simulink model "dq0_fun"  (R2020b)
settings: Solver=FixedStepAuto  StartTime=0.0  StopTime=0.25  FixedStep=1e-3  RelTol=1e-3
libraries: powerlib x13, powerlib_meascontrol x2
settings Model: Creator=kacper  LastModifiedBy=kacper

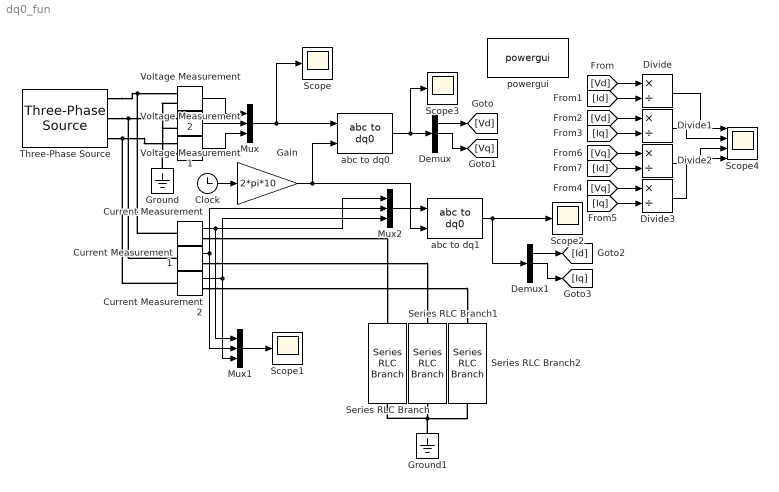
== system dq0_fun ==
  Clock : Clock
  Current Measurement : powerlib/Measurements/Current Measurement  PhasorSimulation=off  OutputType=Complex  PSBequivalent=0
  Current Measurement1 : powerlib/Measurements/Current Measurement  PhasorSimulation=off  OutputType=Complex  PSBequivalent=0
  Current Measurement2 : powerlib/Measurements/Current Measurement  PhasorSimulation=off  OutputType=Complex  PSBequivalent=0
  Demux : Demux  Outputs=3
  Demux1 : Demux  Outputs=3
  Divide{,1..3} (4 alike) : Product  Inputs=*/
  Gain : Gain  Gain=2*pi*10
  Ground : powerlib/Elements/Ground  LConnTagsString=a
  Ground1 : powerlib/Elements/Ground  LConnTagsString=a
  Mux : Mux  Inputs=3
  Mux1 : Mux  Inputs=3
  Mux2 : Mux  Inputs=3
  Scope{,1..3} (4 alike) : Scope
  Scope4 : Scope  NumInputPorts=4
  Series RLC Branch : powerlib/Elements/Series RLC Branch  LConnTagsString=__new0  RConnTagsString=__new0  BranchType=R  Resistance=1  Inductance=1e-3  SetiL0=off  InitialCurrent=0  Capacitance=1e-6  Setx0=off  InitialVoltage=0  Measurements=None
  Series RLC Branch1 : powerlib/Elements/Series RLC Branch  LConnTagsString=__new0  RConnTagsString=__new0  BranchType=L  Resistance=1  Inductance=1  SetiL0=off  InitialCurrent=0  Capacitance=1e-6  Setx0=off  InitialVoltage=0  Measurements=None
  Series RLC Branch2 : powerlib/Elements/Series RLC Branch  LConnTagsString=__new0  RConnTagsString=__new0  BranchType=R  Resistance=1  Inductance=1  SetiL0=off  InitialCurrent=0  Capacitance=1e-6  Setx0=off  InitialVoltage=0  Measurements=None
  Three-Phase Source : powerlib/Electrical Sources/Three-Phase Source  InternalConnection=Yg  VoltagePhases=on  Voltage=1/sqrt(2)  PhaseAngle=0  Voltage_phases=[1/sqrt(2) 1/sqrt(2) 1/sqrt(2)]  PhaseAngles_phases=[0 -120 +120]  Frequency=50  NonIdealSource=off  SpecifyImpedance=off  Resistance=0.8929  Inductance=16.58e-3  ShortCircuitLevel=100e6  BaseVoltage=25e3  XRratio=7  BusType=swing  Pref=10e3  Qref=0  Prefabc=[10e3, 10e3, 10e3]  Qrefabc=[0, 0, 0]  Qmin=-inf  Qmax=inf
  Voltage Measurement : powerlib/Measurements/Voltage Measurement  PhasorSimulation=off  OutputType=Complex  PSBequivalent=0
  Voltage Measurement1 : powerlib/Measurements/Voltage Measurement  PhasorSimulation=off  OutputType=Complex  PSBequivalent=0
  Voltage Measurement2 : powerlib/Measurements/Voltage Measurement  PhasorSimulation=off  OutputType=Complex  PSBequivalent=0
  abc to dq0 : powerlib_meascontrol/Transformations/abc to dq0  Alignment=90 degrees behind phase A axis
  abc to dq1 : powerlib_meascontrol/Transformations/abc to dq0  Alignment=90 degrees behind phase A axis
  powergui : powerlib/powergui  Priority=1  SimulationMode=Continuous  SampleTime=50e-6  frequency=60  Iterations=50  frequencyindice=10  Pbase=100e6  ErrMax=1e-4  UnitsV=kV  UnitsW=MW  buscounter=0  FunctionMessages=off  echomessages=off  EnableUseOfTLC=off  CurrentSourceSwitches=off  DisableSnubberDevices=off  DisableRonSwitches=off  DisableVfSwitches=off  DisplayEquations=off  AutomaticDiscreteSolvers=off  SolverType=Tustin/Backward Euler (TBE)  Interpol=off  ExternalGateDelay=off  methode=off  Ts=100  x0status=blocks  SPID=on  SwTol=0  HookPort=off  NonlinearTolerance=1e-4  nMaxIteration=100  ContinueOnMaxIteration=off  RestoreLinks=warning  ResistiveCurrentMeasurement=off  Frange=[0:2:500]  Ylog=off  Xlog=on  ShowGrid=off  save=off  variable=ZData  structure=0  ZoomFFT=off  StartTime=0.0  cycles=1  DisplayStyle=1  fundamental=60  FreqAxis=off  MaxFrequency=1000  frequencyindicesteady=1  RmsSteady=1  display=off
  wires:
  Voltage Measurement1/1 -> Mux/2
  Voltage Measurement/1 -> Mux/1
  Voltage Measurement2/1 -> Mux/3
  Mux/1 -> Scope/1, abc to dq0/1
  Clock/1 -> Gain/1
  Gain/1 -> abc to dq1/2, abc to dq0/2
  abc to dq0/1 -> Demux/1, Scope3/1
  Mux1/1 -> Scope1/1
  Current Measurement/1 -> Mux2/1, Mux1/1
  Current Measurement1/1 -> Mux2/2, Mux1/2
  Current Measurement2/1 -> Mux2/3, Mux1/3
  Mux2/1 -> abc to dq1/1
  abc to dq1/1 -> Scope2/1, Demux1/1
  Demux/1 -> [Vd]
  Demux/2 -> [Vq]
  Demux1/1 -> [Id]
  Demux1/2 -> [Iq]
  [Vd] -> Divide/1
  [Id] -> Divide/2
  [Iq] -> Divide1/2
  [Vd] -> Divide1/1
  [Iq] -> Divide3/2
  [Vq] -> Divide3/1
  [Id] -> Divide2/2
  [Vq] -> Divide2/1
  Divide/1 -> Scope4/1
  Divide1/1 -> Scope4/2
  Divide2/1 -> Scope4/3
  Divide3/1 -> Scope4/4
  connections:
  Three-Phase Source/RConn1 -- Current Measurement/LConn1 -- Voltage Measurement/LConn1
  Three-Phase Source/RConn2 -- Current Measurement1/LConn1 -- Voltage Measurement1/LConn1
  Three-Phase Source/RConn3 -- Current Measurement2/LConn1 -- Voltage Measurement2/LConn1
  Ground/LConn1 -- Voltage Measurement/LConn2 -- Voltage Measurement1/LConn2 -- Voltage Measurement2/LConn2
  Ground1/LConn1 -- Series RLC Branch1/RConn1 -- Series RLC Branch2/RConn1 -- Series RLC Branch/RConn1
  Current Measurement/RConn1 -- Series RLC Branch/LConn1
  Current Measurement1/RConn1 -- Series RLC Branch1/LConn1
  Current Measurement2/RConn1 -- Series RLC Branch2/LConn1
